simulink model "Heating_System"  (R2015b)
settings: Solver=ode45  StartTime=0.0  StopTime=24  RelTol=1e-3
model workspace (MAT data in the model file):
  M_heater_air = 3600
  R_equivalent = 4.329e-07
  T_heater = 50
  T_roomIC = 20
  c_air = 1005.4
  m_room_air = 1470
settings Model: Creator=Krishnaswamy Kannan  LastModifiedBy=Krishnaswamy Kannan

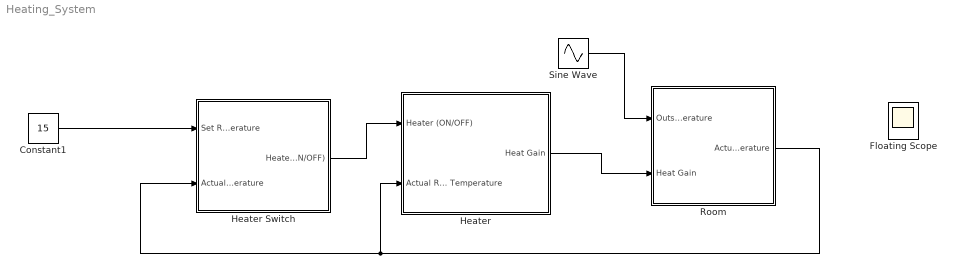
== system Heating_System ==
  Constant1 : Constant  Value=15
  Floating Scope : Scope
      settings: Floating=on
  Heater : Subsystem  TreatAsAtomicUnit=on
  Heater Switch : Subsystem  TreatAsAtomicUnit=on
  Room : Subsystem
  Sine Wave : Sin  Amplitude=5  Bias=12  Frequency=2*pi/24  Phase=180  SampleTime=0
  wires:
  Constant1/1 -> Heater Switch/1(Set Room Temperature)
  Heater Switch/1(Heater (ON/OFF)) -> Heater/1(Heater (ON/OFF))
  Sine Wave/1 -> Room/1(Outside Temperature)
  Heater/1(Heat Gain) -> Room/2("Heat Gain ")
  Room/1("     Actual Room Temperature") -> Heater Switch/2(Actual Room Temperature), Heater/2(Actual Room Temperature)

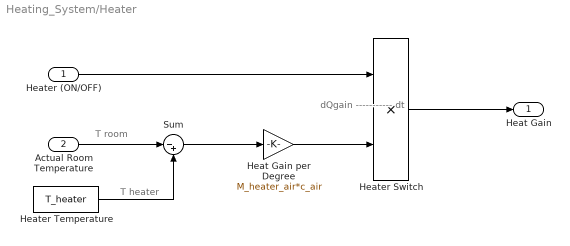
== system Heating_System/Heater ==
  note: dQgain
      | -----------
      |     dt
  note: T heater
  note: T room
  Heater (ON/OFF) : Inport
  Actual Room Temperature : Inport  Port=2
  Heat Gain per Degree : Gain  Gain=M_heater_air*c_air
  Heater Switch : Product
  Heater Temperature : Constant  Value=T_heater
  Sum : Sum  Inputs=|-+
  Heat Gain : Outport
  wires:
  Actual Room Temperature/1 -> Sum/1
  Heater Temperature/1 -> Sum/2
  Sum/1 -> Heat Gain per Degree/1
  Heater (ON/OFF)/1 -> Heater Switch/1
  Heater Switch/1 -> Heat Gain/1
  Heat Gain per Degree/1 -> Heater Switch/2

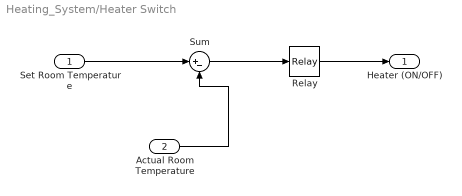
== system Heating_System/Heater Switch ==
  Set Room Temperature : Inport
  Actual Room Temperature : Inport  Port=2
  Relay : Relay  OnSwitchValue=2  OffSwitchValue=-2
  Sum : Sum  Inputs=|+-
  Heater (ON/OFF) : Outport
  wires:
  Set Room Temperature/1 -> Sum/1
  Actual Room Temperature/1 -> Sum/2
  Sum/1 -> Relay/1
  Relay/1 -> Heater (ON/OFF)/1

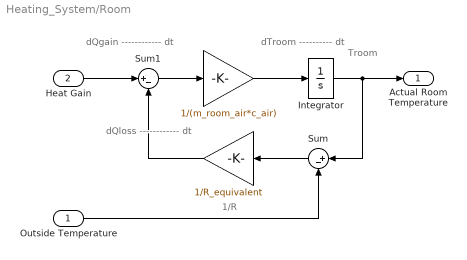
== system Heating_System/Room ==
  note: 1/R
  note: Troom
  note: dQloss
      | ------------
      |      dt
  note: dQgain
      | ------------
      |      dt
  note: dTroom
      | ----------
      |     dt
  Outside Temperature : Inport
  "Heat Gain " : Inport  Port=2
  " " : Gain  Gain=1/R_equivalent  SaturateOnIntegerOverflow=on  OutDataTypeStr=Inherit: Same as input  ParamDataTypeStr=Inherit: Same as input
  "  " : Gain  Gain=1/(m_room_air*c_air)  SaturateOnIntegerOverflow=on  OutDataTypeStr=Inherit: Same as input  ParamDataTypeStr=Inherit: Same as input
  Integrator : Integrator  InitialCondition=T_roomIC
  Sum : Sum  Inputs=|+-
  Sum1 : Sum  Inputs=|+-  SaturateOnIntegerOverflow=on  InputSameDT=on  OutDataTypeStr=Inherit: Same as first input
  "     Actual Room Temperature" : Outport
  wires:
  "Heat Gain "/1 -> Sum1/1
  Sum1/1 -> "  "/1
  "  "/1 -> Integrator/1
  Integrator/1 -> Sum/1, "     Actual Room Temperature"/1
  " "/1 -> Sum1/2
  Sum/1 -> " "/1
  Outside Temperature/1 -> Sum/2
